simulink model "massspringsystem"  (R2015b)
settings: Solver=ode23tb  StartTime=0.0  StopTime=100  RelTol=1e-3
values from neighbouring files (symbols this model uses):
  B = 30    [cruise_speed.m]    (also in mass_spring.m = 15; parameter_values.m)
  F = 300    [parameter_values.m]
  K = 15    [mass_spring.m]    (also in parameter_values.m)
  M = 750    [cruise_speed.m]    (also in mass_spring.m; parameter_values.m)
settings Model: Creator=Arshad  LastModifiedBy=Sir Arshad
settings DataIOCC: SaveFormat=Array  SignalLoggingSaveFormat=ModelDataLogs
settings OptimizationCC: ExpressionDepthLimit=2147483647
settings DebuggingCC: UnderspecifiedInitializationDetection=Classic  MergeDetectMultiDrivingBlocksExec=none  SolverPrmCheckMsg=warning  FcnCallInpInsideContextMsg=UseLocalSettings  StateNameClashWarn=warning
settings HardwareCC: ProdBitPerPointer=32  ProdLargestAtomicFloat=None  ProdIntDivRoundTo=Undefined  ProdEndianess=Unspecified  ProdWordSize=32  ProdHWDeviceType=32-bit Generic
settings GRTTargetCC: GeneratePreprocessorConditionals=Disable all  CombineOutputUpdateFcns=off  GRTInterface=on

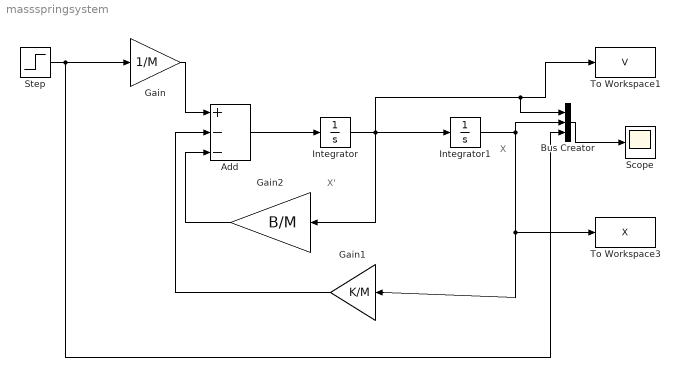
== system massspringsystem ==
  note: X'
  note: X
  Add : Sum  Inputs=+--
  Bus Creator : BusCreator  Inputs=3
  Gain : Gain  Gain=1/M
  Gain1 : Gain  Gain=K/M
  Gain2 : Gain  Gain=B/M
  Integrator : Integrator
  Integrator1 : Integrator
  Scope : Scope
  Step : Step  Time=0  After=F  SampleTime=0
  To Workspace1 : ToWorkspace  VariableName=V  SampleTime=-1
  To Workspace3 : ToWorkspace  VariableName=X  SampleTime=-1
  wires:
  Gain/1 -> Add/1
  Add/1 -> Integrator/1
  Integrator/1 -> Integrator1/1, Gain2/1, To Workspace1/1, Bus Creator/1
  Gain2/1 -> Add/3
  Integrator1/1 -> Gain1/1, To Workspace3/1, Bus Creator/2
  Gain1/1 -> Add/2
  Bus Creator/1 -> Scope/1
  Step/1 -> Gain/1, Bus Creator/3
